simulink model "observer_mass"  (R2021a)
settings: Solver=VariableStepAuto  StartTime=0.0  StopTime=50  RelTol=1e-3
values from neighbouring files (symbols this model uses):
  c = 1    [init_graph.m]
  F = F'    [init_graph.m]
undefined symbols (not defined in the file or in its folder): A, B, C, D, D_o, K
settings Model: Creator=umut  LastModifiedBy=umut

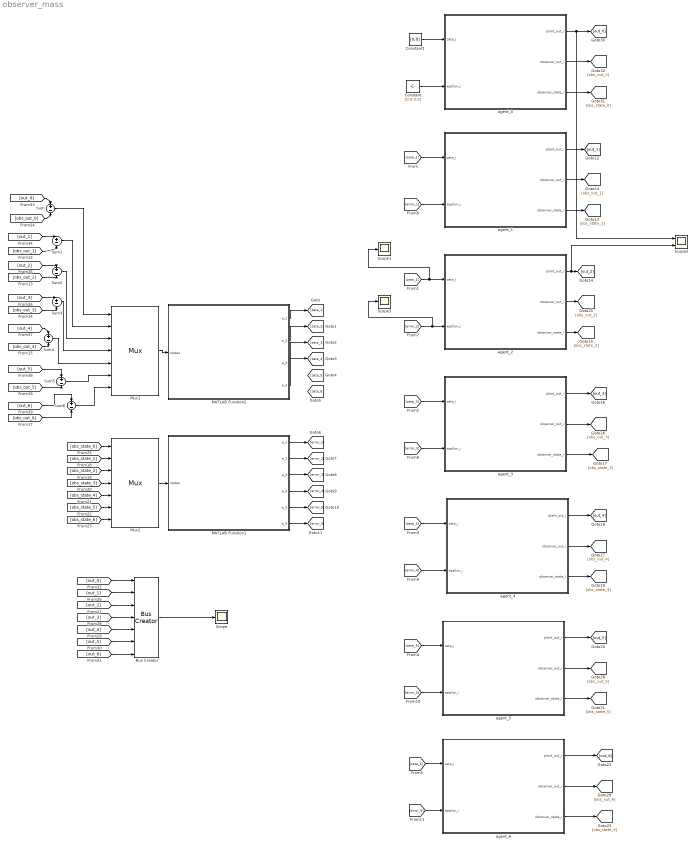
== system observer_mass ==
  Bus Creator : BusCreator  Inputs=7
  Constant : Constant  Value=[0;0;0;0]
  Constant1 : Constant  Value=[0;0]
  MATLAB Function1 : MATLAB Function  TreatAsAtomicUnit=on
  MATLAB Function2 : MATLAB Function  TreatAsAtomicUnit=on
  Mux1 : Mux  Inputs=7
  Mux2 : Mux  Inputs=7
  Scope : Scope
  Scope1 : Scope
  Scope2 : Scope  NumInputPorts=2
  Scope3 : Scope
  Sum{,1..6} (7 alike) : Sum  Inputs=+|-
  agent_0 : Subsystem
  agent_1 : Subsystem
  agent_2 : Subsystem
  agent_3 : Subsystem
  agent_4 : Subsystem
  agent_5 : Subsystem
  agent_6 : Subsystem
  wires:
  MATLAB Function2/1(e_1) -> [zeta_1]
  MATLAB Function2/2(e_2) -> [zeta_2]
  MATLAB Function2/4(e_4) -> [zeta_4]
  MATLAB Function2/3(e_3) -> [zeta_3]
  ? -> [zeta_5]
  ? -> [zeta_6]
  MATLAB Function1/3(e_3) -> [error_3]
  MATLAB Function1/5(e_5) -> [error_5]
  MATLAB Function1/2(e_2) -> [error_2]
  MATLAB Function1/1(e_1) -> [error_1]
  MATLAB Function1/4(e_4) -> [error_4]
  MATLAB Function1/6(e_6) -> [error_6]
  [zeta_3] -> agent_3/1(zeta_i)
  [zeta_2] -> Scope1/1, agent_2/1(zeta_i)
  [zeta_4] -> agent_4/1(zeta_i)
  [zeta_5] -> agent_5/1(zeta_i)
  [zeta_6] -> agent_6/1(zeta_i)
  [error_3] -> agent_3/2(epsilon_i)
  [error_4] -> agent_4/2(epsilon_i)
  [error_5] -> agent_5/2(epsilon_i)
  [error_2] -> Scope3/1, agent_2/2(epsilon_i)
  [error_6] -> agent_6/2(epsilon_i)
  agent_1/1(plant_out_i) -> [out_1]
  agent_1/3(observer_state_i) -> [obs_state_1]
  agent_2/1(plant_out_i) -> Scope2/2, [out_2]
  agent_2/3(observer_state_i) -> [obs_state_2]
  agent_3/1(plant_out_i) -> [out_3]
  agent_3/3(observer_state_i) -> [obs_state_3]
  agent_4/1(plant_out_i) -> [out_4]
  agent_4/3(observer_state_i) -> [obs_state_4]
  agent_5/1(plant_out_i) -> [out_5]
  agent_5/3(observer_state_i) -> [obs_state_5]
  agent_6/1(plant_out_i) -> [out_6]
  agent_6/3(observer_state_i) -> [obs_state_6]
  Mux1/1 -> MATLAB Function2/1(states)
  Sum1/1 -> Mux1/2
  Sum2/1 -> Mux1/3
  Sum3/1 -> Mux1/4
  Sum4/1 -> Mux1/5
  Sum5/1 -> Mux1/6
  Sum6/1 -> Mux1/7
  agent_1/2(observer_out_i) -> [obs_out_1]
  agent_2/2(observer_out_i) -> [obs_out_2]
  agent_3/2(observer_out_i) -> [obs_out_3]
  agent_4/2(observer_out_i) -> [obs_out_4]
  agent_5/2(observer_out_i) -> [obs_out_5]
  agent_6/2(observer_out_i) -> [obs_out_6]
  [obs_state_4] -> Mux2/5
  [obs_state_5] -> Mux2/6
  [obs_state_2] -> Mux2/3
  [obs_state_6] -> Mux2/7
  [obs_state_3] -> Mux2/4
  [obs_state_1] -> Mux2/2
  Mux2/1 -> MATLAB Function1/1(states)
  [error_1] -> agent_1/2(epsilon_i)
  [zeta_1] -> agent_1/1(zeta_i)
  agent_0/2(observer_out_i) -> [obs_out_0]
  agent_0/3(observer_state_i) -> [obs_state_0]
  Sum/1 -> Mux1/1
  [obs_state_0] -> Mux2/1
  [out_0] -> Bus Creator/1
  [out_1] -> Bus Creator/2
  [out_2] -> Bus Creator/3
  [out_3] -> Bus Creator/4
  [out_4] -> Bus Creator/5
  [out_5] -> Bus Creator/6
  [out_6] -> Bus Creator/7
  Bus Creator/1 -> Scope/1
  Constant1/1 -> agent_0/1(zeta_i)
  Constant/1 -> agent_0/2(epsilon_i)
  agent_0/1(plant_out_i) -> Scope2/1, [out_0]
  [obs_out_0] -> Sum/2
  [out_0] -> Sum/1
  [obs_out_1] -> Sum1/2
  [out_1] -> Sum1/1
  [obs_out_2] -> Sum2/2
  [out_2] -> Sum2/1
  [obs_out_3] -> Sum3/2
  [out_3] -> Sum3/1
  [out_4] -> Sum4/1
  [obs_out_4] -> Sum4/2
  [out_5] -> Sum5/1
  [obs_out_5] -> Sum5/2
  [out_6] -> Sum6/1
  [obs_out_6] -> Sum6/2

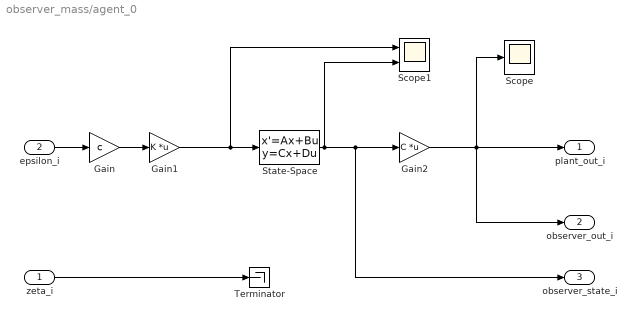
== system observer_mass/agent_0 ==
  zeta_i : Inport
  epsilon_i : Inport  Port=2
  Gain : Gain  Gain=c
  Gain1 : Gain  Gain=K  Multiplication=Matrix(K*u)
  Gain2 : Gain  Gain=C  Multiplication=Matrix(K*u)
  Scope : Scope
  Scope1 : Scope  NumInputPorts=2
  State-Space : StateSpace  A=A  B=B  C=eye(4)  D=D  InitialCondition=[1;2;3;4]
  Terminator : Terminator
  plant_out_i : Outport
  observer_out_i : Outport  Port=2
  observer_state_i : Outport  Port=3
  wires:
  epsilon_i/1 -> Gain/1
  zeta_i/1 -> Terminator/1
  Gain/1 -> Gain1/1
  Gain1/1 -> Scope1/1, State-Space/1
  Gain2/1 -> Scope/1, plant_out_i/1, observer_out_i/1
  State-Space/1 -> Scope1/2, observer_state_i/1, Gain2/1

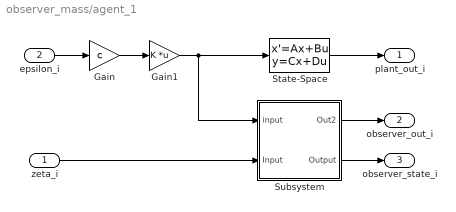
== system observer_mass/agent_1 ==
  zeta_i : Inport
  epsilon_i : Inport  Port=2
  Gain : Gain  Gain=c
  Gain1 : Gain  Gain=K  Multiplication=Matrix(K*u)
  State-Space : StateSpace  A=A  B=B  C=C  D=D_o  InitialCondition=[1;2;3;4]
  Subsystem : Subsystem
  plant_out_i : Outport
  observer_out_i : Outport  Port=2
  observer_state_i : Outport  Port=3
  wires:
  epsilon_i/1 -> Gain/1
  State-Space/1 -> plant_out_i/1
  Subsystem/1(Out2) -> observer_out_i/1
  Subsystem/2(Output) -> observer_state_i/1
  zeta_i/1 -> Subsystem/2(Input)
  Gain/1 -> Gain1/1
  Gain1/1 -> State-Space/1, Subsystem/1(input)

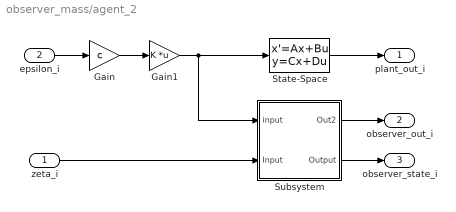
== system observer_mass/agent_2 ==
  zeta_i : Inport
  epsilon_i : Inport  Port=2
  Gain : Gain  Gain=c
  Gain1 : Gain  Gain=K  Multiplication=Matrix(K*u)
  State-Space : StateSpace  A=A  B=B  C=C  D=D_o  InitialCondition=[2;3;4;5]
  Subsystem : Subsystem
  plant_out_i : Outport
  observer_out_i : Outport  Port=2
  observer_state_i : Outport  Port=3
  wires:
  epsilon_i/1 -> Gain/1
  State-Space/1 -> plant_out_i/1
  Subsystem/1(Out2) -> observer_out_i/1
  Subsystem/2(Output) -> observer_state_i/1
  zeta_i/1 -> Subsystem/2(Input)
  Gain/1 -> Gain1/1
  Gain1/1 -> State-Space/1, Subsystem/1(input)

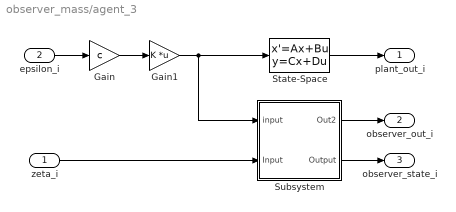
== system observer_mass/agent_3 ==
  zeta_i : Inport
  epsilon_i : Inport  Port=2
  Gain : Gain  Gain=c
  Gain1 : Gain  Gain=K  Multiplication=Matrix(K*u)
  State-Space : StateSpace  A=A  B=B  C=C  D=D_o  InitialCondition=[1;2;3;4]
  Subsystem : Subsystem
  plant_out_i : Outport
  observer_out_i : Outport  Port=2
  observer_state_i : Outport  Port=3
  wires:
  epsilon_i/1 -> Gain/1
  State-Space/1 -> plant_out_i/1
  Subsystem/1(Out2) -> observer_out_i/1
  Subsystem/2(Output) -> observer_state_i/1
  zeta_i/1 -> Subsystem/2(Input)
  Gain/1 -> Gain1/1
  Gain1/1 -> State-Space/1, Subsystem/1(input)

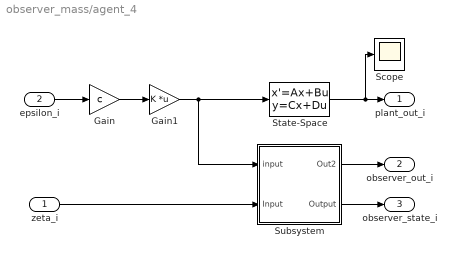
== system observer_mass/agent_4 ==
  zeta_i : Inport
  epsilon_i : Inport  Port=2
  Gain : Gain  Gain=c
  Gain1 : Gain  Gain=K  Multiplication=Matrix(K*u)
  Scope : Scope
  State-Space : StateSpace  A=A  B=B  C=C  D=D_o  InitialCondition=[1;2;3;4]
  Subsystem : Subsystem
  plant_out_i : Outport
  observer_out_i : Outport  Port=2
  observer_state_i : Outport  Port=3
  wires:
  epsilon_i/1 -> Gain/1
  State-Space/1 -> Scope/1, plant_out_i/1
  Subsystem/1(Out2) -> observer_out_i/1
  Subsystem/2(Output) -> observer_state_i/1
  zeta_i/1 -> Subsystem/2(Input)
  Gain/1 -> Gain1/1
  Gain1/1 -> State-Space/1, Subsystem/1(input)

== system observer_mass/agent_5 ==
  zeta_i : Inport
  epsilon_i : Inport  Port=2
  Gain : Gain  Gain=c
  Gain1 : Gain  Gain=K  Multiplication=Matrix(K*u)
  State-Space : StateSpace  A=A  B=B  C=C  D=D_o  InitialCondition=[1;2;3;4]
  Subsystem : Subsystem
  plant_out_i : Outport
  observer_out_i : Outport  Port=2
  observer_state_i : Outport  Port=3
  wires:
  epsilon_i/1 -> Gain/1
  State-Space/1 -> plant_out_i/1
  Subsystem/1(Out2) -> observer_out_i/1
  Subsystem/2(Output) -> observer_state_i/1
  zeta_i/1 -> Subsystem/2(Input)
  Gain/1 -> Gain1/1
  Gain1/1 -> State-Space/1, Subsystem/1(input)

== system observer_mass/agent_6 ==
  zeta_i : Inport
  epsilon_i : Inport  Port=2
  Gain : Gain  Gain=c
  Gain1 : Gain  Gain=K  Multiplication=Matrix(K*u)
  State-Space : StateSpace  A=A  B=B  C=C  D=D_o  InitialCondition=[1;2;3;4]
  Subsystem : Subsystem
  plant_out_i : Outport
  observer_out_i : Outport  Port=2
  observer_state_i : Outport  Port=3
  wires:
  epsilon_i/1 -> Gain/1
  State-Space/1 -> plant_out_i/1
  Subsystem/1(Out2) -> observer_out_i/1
  Subsystem/2(Output) -> observer_state_i/1
  zeta_i/1 -> Subsystem/2(Input)
  Gain/1 -> Gain1/1
  Gain1/1 -> State-Space/1, Subsystem/1(input)

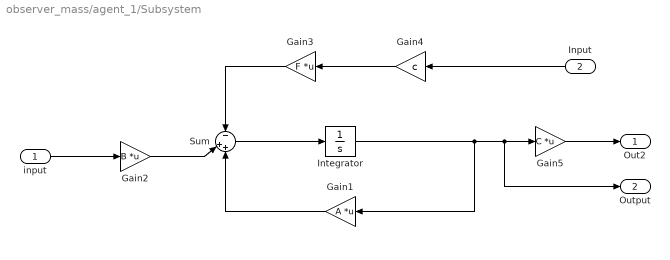
== system observer_mass/agent_1/Subsystem ==
  input : Inport
  Input : Inport  Port=2
  Gain1 : Gain  Gain=A  Multiplication=Matrix(K*u)
  Gain2 : Gain  Gain=B  Multiplication=Matrix(K*u)
  Gain3 : Gain  Gain=F  Multiplication=Matrix(K*u)
  Gain4 : Gain  Gain=c
  Gain5 : Gain  Gain=C  Multiplication=Matrix(K*u)
  Integrator : Integrator
  Sum : Sum  Inputs=-|++
  Out2 : Outport
  Output : Outport  Port=2
  wires:
  Gain3/1 -> Sum/1
  Gain2/1 -> Sum/2
  input/1 -> Gain2/1
  Gain1/1 -> Sum/3
  Sum/1 -> Integrator/1
  Gain5/1 -> Out2/1
  Input/1 -> Gain4/1
  Gain4/1 -> Gain3/1
  Integrator/1 -> Output/1, Gain5/1, Gain1/1

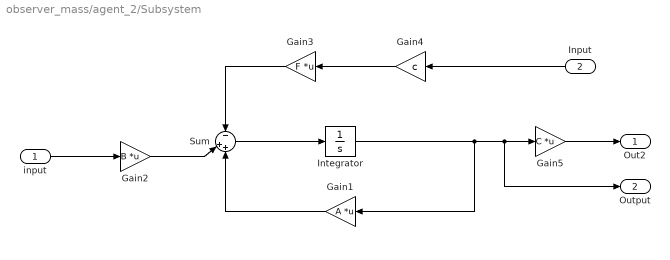
== system observer_mass/agent_2/Subsystem ==
  input : Inport
  Input : Inport  Port=2
  Gain1 : Gain  Gain=A  Multiplication=Matrix(K*u)
  Gain2 : Gain  Gain=B  Multiplication=Matrix(K*u)
  Gain3 : Gain  Gain=F  Multiplication=Matrix(K*u)
  Gain4 : Gain  Gain=c
  Gain5 : Gain  Gain=C  Multiplication=Matrix(K*u)
  Integrator : Integrator
  Sum : Sum  Inputs=-|++
  Out2 : Outport
  Output : Outport  Port=2
  wires:
  Gain3/1 -> Sum/1
  Gain2/1 -> Sum/2
  input/1 -> Gain2/1
  Gain1/1 -> Sum/3
  Sum/1 -> Integrator/1
  Gain5/1 -> Out2/1
  Input/1 -> Gain4/1
  Gain4/1 -> Gain3/1
  Integrator/1 -> Output/1, Gain5/1, Gain1/1

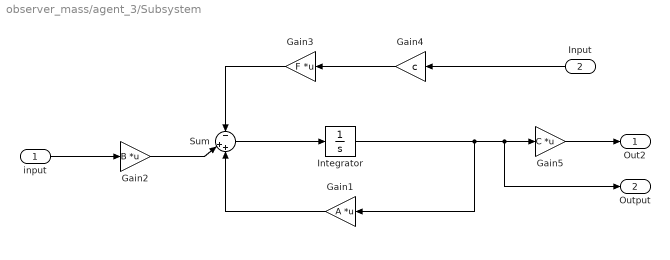
== system observer_mass/agent_3/Subsystem ==
  input : Inport
  Input : Inport  Port=2
  Gain1 : Gain  Gain=A  Multiplication=Matrix(K*u)
  Gain2 : Gain  Gain=B  Multiplication=Matrix(K*u)
  Gain3 : Gain  Gain=F  Multiplication=Matrix(K*u)
  Gain4 : Gain  Gain=c
  Gain5 : Gain  Gain=C  Multiplication=Matrix(K*u)
  Integrator : Integrator
  Sum : Sum  Inputs=-|++
  Out2 : Outport
  Output : Outport  Port=2
  wires:
  Gain3/1 -> Sum/1
  Gain2/1 -> Sum/2
  input/1 -> Gain2/1
  Gain1/1 -> Sum/3
  Sum/1 -> Integrator/1
  Gain5/1 -> Out2/1
  Input/1 -> Gain4/1
  Gain4/1 -> Gain3/1
  Integrator/1 -> Output/1, Gain5/1, Gain1/1

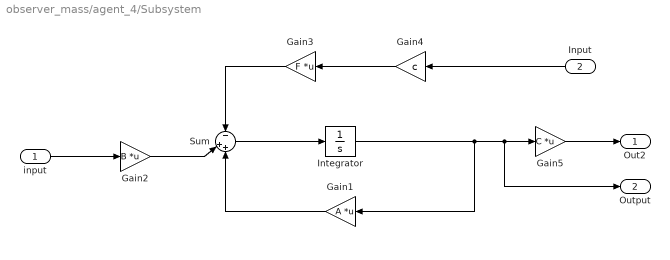
== system observer_mass/agent_4/Subsystem ==
  input : Inport
  Input : Inport  Port=2
  Gain1 : Gain  Gain=A  Multiplication=Matrix(K*u)
  Gain2 : Gain  Gain=B  Multiplication=Matrix(K*u)
  Gain3 : Gain  Gain=F  Multiplication=Matrix(K*u)
  Gain4 : Gain  Gain=c
  Gain5 : Gain  Gain=C  Multiplication=Matrix(K*u)
  Integrator : Integrator
  Sum : Sum  Inputs=-|++
  Out2 : Outport
  Output : Outport  Port=2
  wires:
  Gain3/1 -> Sum/1
  Gain2/1 -> Sum/2
  input/1 -> Gain2/1
  Gain1/1 -> Sum/3
  Sum/1 -> Integrator/1
  Gain5/1 -> Out2/1
  Input/1 -> Gain4/1
  Gain4/1 -> Gain3/1
  Integrator/1 -> Output/1, Gain5/1, Gain1/1

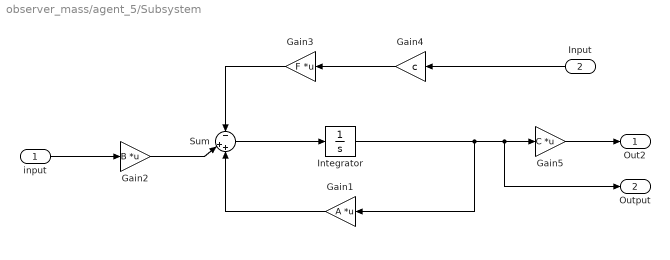
== system observer_mass/agent_5/Subsystem ==
  input : Inport
  Input : Inport  Port=2
  Gain1 : Gain  Gain=A  Multiplication=Matrix(K*u)
  Gain2 : Gain  Gain=B  Multiplication=Matrix(K*u)
  Gain3 : Gain  Gain=F  Multiplication=Matrix(K*u)
  Gain4 : Gain  Gain=c
  Gain5 : Gain  Gain=C  Multiplication=Matrix(K*u)
  Integrator : Integrator
  Sum : Sum  Inputs=-|++
  Out2 : Outport
  Output : Outport  Port=2
  wires:
  Gain3/1 -> Sum/1
  Gain2/1 -> Sum/2
  input/1 -> Gain2/1
  Gain1/1 -> Sum/3
  Sum/1 -> Integrator/1
  Gain5/1 -> Out2/1
  Input/1 -> Gain4/1
  Gain4/1 -> Gain3/1
  Integrator/1 -> Output/1, Gain5/1, Gain1/1

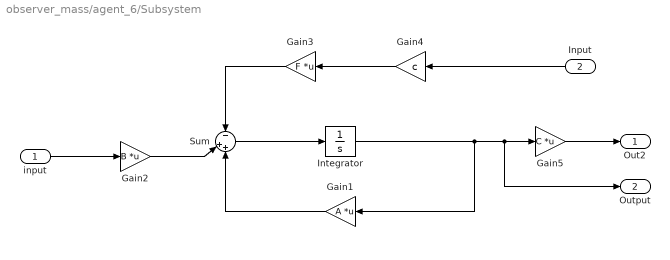
== system observer_mass/agent_6/Subsystem ==
  input : Inport
  Input : Inport  Port=2
  Gain1 : Gain  Gain=A  Multiplication=Matrix(K*u)
  Gain2 : Gain  Gain=B  Multiplication=Matrix(K*u)
  Gain3 : Gain  Gain=F  Multiplication=Matrix(K*u)
  Gain4 : Gain  Gain=c
  Gain5 : Gain  Gain=C  Multiplication=Matrix(K*u)
  Integrator : Integrator
  Sum : Sum  Inputs=-|++
  Out2 : Outport
  Output : Outport  Port=2
  wires:
  Gain3/1 -> Sum/1
  Gain2/1 -> Sum/2
  input/1 -> Gain2/1
  Gain1/1 -> Sum/3
  Sum/1 -> Integrator/1
  Gain5/1 -> Out2/1
  Input/1 -> Gain4/1
  Gain4/1 -> Gain3/1
  Integrator/1 -> Output/1, Gain5/1, Gain1/1

== matlab function observer_mass/MATLAB Function1 ==
  data: states input; e_1 output size=[4, 1]; e_2 output size=[4, 1]; e_3 output size=[4, 1]; e_4 output size=[4, 1]; e_5 output size=[4, 1]; e_6 output size=[4, 1]
function [e_1, e_2, e_3, e_4, e_5, e_6]  = calculate_neighborhood_error(states)
    adj = [ 0	0	0	0	0	0
        2	0	0	0	0	0
        0	6	0	0	0	0
        0	0	1	0	0	0
        0	0	0	1	0	0
        0	0	0	0	3	0];
    
    pinnings = [1; 0; 0; 0; 0; 0];

    A = adj;
    G = pinnings;
    
    size_agents = 6;
    size_states = 4;
    
    error = zeros(size_states, size_agents);
    
    
    for i = 1 : size_agents
        error_temp = [0;0;0;0];
        for j = 1 : size_agents
            error_temp = error_temp + A(i, j) * (states((j)*4+1 : 4*(j+1)) - states((i)*4+1 : 4*(i+1)));
        end
        error_temp = error_temp + pinnings(i) * (states(1 : 4) - states((i)*4+1 : 4*(i+1)));
        error(:,i) = error_temp;
    end
    
    e_1 = error(:,1);
    e_2 = error(:,2);
    e_3 = error(:,3);
    e_4 = error(:,4);
    e_5 = error(:,5);
    e_6 = error(:,6);

end

== matlab function observer_mass/MATLAB Function2 ==
  data: states input; e_1 output size=[2, 1]; e_2 output size=[2, 1]; e_3 output size=[2, 1]; e_4 output size=[2, 1]
function [e_1, e_2, e_3, e_4]  = calculate_output_error(states)
    adj_o = [ 0	0	0	0	0	0
        2	0	0	0	0	0
        0	6	0	0	0	0
        0	0	1	0	0	0
        0	0	0	1	0	0
        0	0	0	0	3	0];    
    
    pinnings = [1; 0; 0; 0; 0; 0];

    A = adj_o;
    G = pinnings;
    
    size_agents = 4;
    size_states = 2;
    
    error = zeros(size_states, size_agents);
    
    
    for i = 1 : size_agents
        error_temp = [0;0];
        for j = 1 : size_agents
            error_temp = error_temp + A(i, j) * (states((j)*size_states+1 : size_states*(j+1)) - states((i)*size_states+1 : size_states*(i+1)));
        end
        error_temp = error_temp + pinnings(i) * (states(1 : size_states) - states((i)*size_states+1 : size_states*(i+1)));
        error(:,i) = error_temp;
    end
    
    e_1 = error(:,1);
    e_2 = error(:,2);
    e_3 = error(:,3);
    e_4 = error(:,4);
end
